simulink model "corBF"  (R2016b)
settings: Solver=VariableStepAuto  StartTime=0.0  StopTime=10.0  RelTol=1e-3
values from neighbouring files (symbols this model uses):
  f = 120    [Cons.m]
  Kconv = 7.576    [Cons.m]
  Ki = 43.2/1000    (= 0.0432)    [Cons.m]
  Kred = 35.9    [Cons.m]
  meq = 120    [Cons.m]
  rpignon = 21*0.8/(2*1000)    (= 0.0084)    [Cons.m]
settings Model: Creator=emilien.durif  LastModifiedBy=emilien.durif

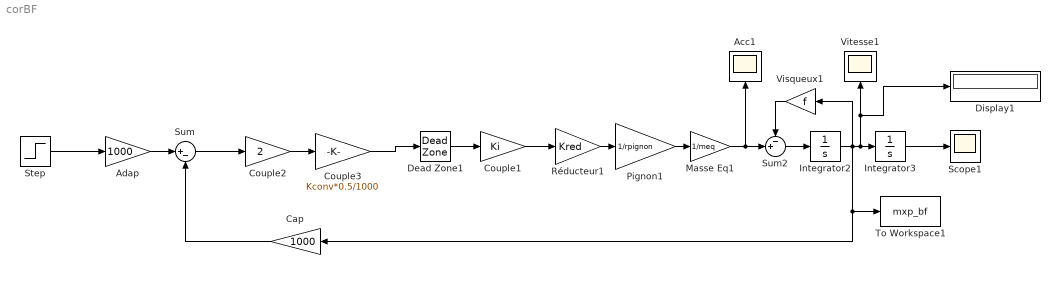
== system corBF ==
  Acc1 : Scope
  Adap : Gain  Gain=1000
  Cap : Gain  Gain=1000
  Couple1 : Gain  Gain=Ki
  Couple2 : Gain  Gain=2
  Couple3 : Gain  Gain=Kconv*0.5/1000
  Dead Zone1 : DeadZone  LowerValue=-0.05  UpperValue=0.05  SaturateOnIntegerOverflow=on
  Display1 : Display
  Integrator2 : Integrator
  Integrator3 : Integrator
  Masse Eq1 : Gain  Gain=1/meq
  Pignon1 : Gain  Gain=1/rpignon
  Réducteur1 : Gain  Gain=Kred
  Scope1 : Scope
  Step : Step  Time=0.1  After=0.1  SampleTime=0
  Sum : Sum  Inputs=|+-
  Sum2 : Sum  Inputs=-+|
  To Workspace1 : ToWorkspace  VariableName=mxp_bf  SaveFormat=Timeseries  SampleTime=-1
  Visqueux1 : Gain  Gain=f
  Vitesse1 : Scope
  wires:
  Step/1 -> Adap/1
  Adap/1 -> Sum/1
  Cap/1 -> Sum/2
  Pignon1/1 -> Masse Eq1/1
  Integrator2/1 -> To Workspace1/1, Cap/1, Visqueux1/1, Display1/1, Vitesse1/1, Integrator3/1
  Integrator3/1 -> Scope1/1
  Sum2/1 -> Integrator2/1
  Visqueux1/1 -> Sum2/1
  Masse Eq1/1 -> Sum2/2, Acc1/1
  Réducteur1/1 -> Pignon1/1
  Couple1/1 -> Réducteur1/1
  Sum/1 -> Couple2/1
  Couple2/1 -> Couple3/1
  Dead Zone1/1 -> Couple1/1
  Couple3/1 -> Dead Zone1/1
